simulink model "Events2"  (Simulink 5.0)
settings: Solver=ode45  StartTime=0.0  StopTime=10.0  RelTol=1e-3
settings Model: Creator=scaife  LastModifiedBy=scaife  ExtModeAutoUpdateStatusClock=off

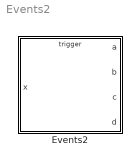
== system Events2 ==
  Events2 : Stateflow chart

== stateflow chart Events2 ==
  state B [parallel]
    state Ba/
      en:b=x+3
    state Bb/
      en:b=x+4
    (default) -> Ba
    Bb -> Ba : R1/R2
    Ba -> Bb : S1/S2
  state A [parallel]
    state Aa/
      en:a=x+1
    state Ab/
      en:a=x+2
    (default) -> Aa
    Aa -> Ab : S/S1
    Ab -> Aa : R/R1
  state D [parallel]
    state Da/
      en:d=x+7
    state Db/
      en:d=x+8
    Db -> Da : R3
    (default) -> Da
    Da -> Db : S3
  state C [parallel]
    state Cb/
      en:c=x+6
    state Ca/
      en:c=x+5
    Ca -> Cb : S2/S3
    Cb -> Ca : R2/R3
    (default) -> Ca
  data: a output int32; x input int32; b output int32; c output int32; d output int32
  events: R1 local EITHER_EDGE_EVENT; S1 local EITHER_EDGE_EVENT; R input EITHER_EDGE_EVENT; S input EITHER_EDGE_EVENT; R2 local EITHER_EDGE_EVENT; S2 local EITHER_EDGE_EVENT; S3 local EITHER_EDGE_EVENT; R3 local EITHER_EDGE_EVENT
